simulink model "testSim"  (R2019a)
settings: Solver=VariableStepAuto  StartTime=0.0  StopTime=10.0  RelTol=1e-3
settings Model: Creator=magneasi  LastModifiedBy=magneasi

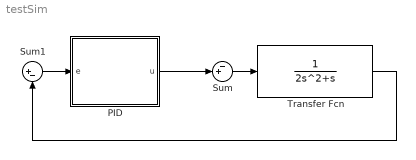
== system testSim ==
  PID : Subsystem  mask{Kp=0, Ki=0, Kd=0}
  Sum : Sum  Inputs=-+|
  Sum1 : Sum  Inputs=|+-
  Transfer Fcn : TransferFcn  Denominator=[2 1 0]
  wires:
  PID/1("u ") -> Sum/2
  Sum/1 -> Transfer Fcn/1
  ? -> Sum/1
  Sum1/1 -> PID/1(e)
  Transfer Fcn/1 -> Sum1/2
  ? -> Sum1/1

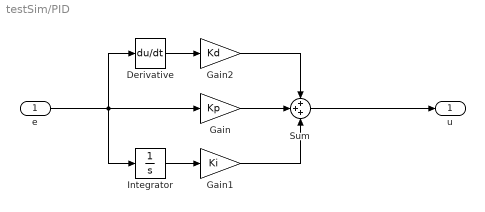
== system testSim/PID ==
  e : Inport
  Derivative : Derivative
  Gain : Gain  Gain=Kp
  Gain1 : Gain  Gain=Ki
  Gain2 : Gain  Gain=Kd
  Integrator : Integrator
  Sum : Sum  Inputs=+++
  "u " : Outport
  wires:
  Derivative/1 -> Gain2/1
  Gain/1 -> Sum/2
  Gain1/1 -> Sum/3
  Sum/1 -> "u "/1
  Gain2/1 -> Sum/1
  e/1 -> Integrator/1, Derivative/1, Gain/1
  Integrator/1 -> Gain1/1
